simulink model "ex3"  (Simulink 6.3)
settings: Solver=VariableStepDiscrete  StartTime=0.0  StopTime=10  RelTol=1e-3
values from neighbouring files (symbols this model uses):
  SymbolRate = 50000    [ex3sim.m]
undefined symbols (not defined in the file or in its folder): gfprimfd
libraries: commdigbbndpm2 x4, dspbuff3 x3, commchan3 x2, commsink2 x2, commblkcod2 x2, dspsigops x1, commrandsrc2 x1
settings Model: LastModifiedBy=lxy  StrictBusMsg=None
settings OptimizationCC: InlineInvariantSignals=on

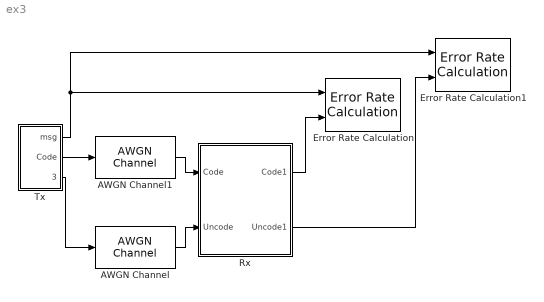
== system ex3 ==
  AWGN Channel : commchan3/AWGN Channel  seed=12345  noiseMode="Signal to noise ratio  (Eb/No)"  EbNodB=SNR  EsNodB=10  SNRdB=10  bitsPerSym=2  Ps=1  Tsym=1/SymbolRate  variance=1
  AWGN Channel1 : commchan3/AWGN Channel  seed=12345  noiseMode="Signal to noise ratio  (Eb/No)"  EbNodB=SNR  EsNodB=10  SNRdB=10  bitsPerSym=2  Ps=1  Tsym=1/SymbolRate  variance=1
  Error Rate Calculation : commsink2/Error Rate Calculation  N=8  st_delay=0  cp_mode=Entire frame  subframe=[]  PMode=Workspace  WsName=BER2  RsMode2=off  stop=off  numErr=100  maxBits=1e6
  Error Rate Calculation1 : commsink2/Error Rate Calculation  N=0  st_delay=0  cp_mode=Entire frame  subframe=[]  PMode=Workspace  WsName=BER1  RsMode2=off  stop=off  numErr=100  maxBits=1e6
  Rx : Subsystem
  Tx : Subsystem
  wires:
  Tx/2(Code) -> AWGN Channel1/1
  Tx/3(Uncode) -> AWGN Channel/1
  AWGN Channel/1 -> Rx/2(Uncode)
  AWGN Channel1/1 -> Rx/1(Code)
  Tx/1(msg) -> Error Rate Calculation/1, Error Rate Calculation1/1
  Rx/1(Code1) -> Error Rate Calculation/2
  Rx/2(Uncode1) -> Error Rate Calculation1/2

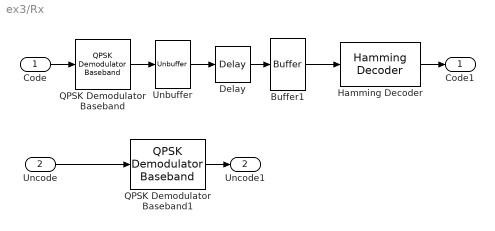
== system ex3/Rx ==
  Code : Inport
  Uncode : Inport  Port=2
  Buffer1 : dspbuff3/Buffer  N=7  V=0  ic=4
  Delay : dspsigops/Delay  dly_unit=Samples  delay=5  ic_detail=off  dif_ic_for_ch=off  dif_ic_for_dly=off  ic=0  reset_popup=None
  Hamming Decoder : commblkcod2/Hamming Decoder  n=7  k=gfprimfd(3,'min')
  QPSK Demodulator Baseband : commdigbbndpm2/QPSK Demodulator Baseband  OutType=Bit  Dec=Gray  Ph=pi/4  numSamp=1
  QPSK Demodulator Baseband1 : commdigbbndpm2/QPSK Demodulator Baseband  OutType=Bit  Dec=Gray  Ph=pi/4  numSamp=1
  Unbuffer : dspbuff3/Unbuffer  ic=0
  Code1 : Outport
  Uncode1 : Outport  Port=2
  wires:
  Hamming Decoder/1 -> Code1/1
  Code/1 -> QPSK Demodulator Baseband/1
  Uncode/1 -> QPSK Demodulator Baseband1/1
  QPSK Demodulator Baseband1/1 -> Uncode1/1
  QPSK Demodulator Baseband/1 -> Unbuffer/1
  Unbuffer/1 -> Delay/1
  Delay/1 -> Buffer1/1
  Buffer1/1 -> Hamming Decoder/1

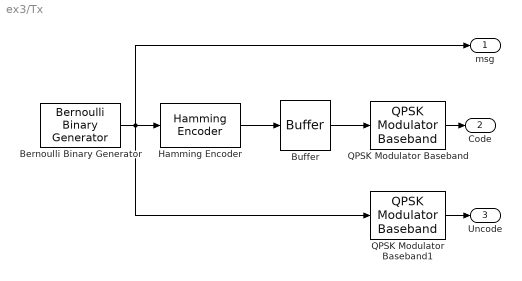
== system ex3/Tx ==
  Bernoulli Binary Generator : commrandsrc2/Bernoulli Binary Generator  P=0.5  seed=61  Ts=1/(2*SymbolRate)  frameBased=on  sampPerFrame=4  orient=off  outDataType=double
  Buffer : dspbuff3/Buffer  N=2  V=0  ic=0
  Hamming Encoder : commblkcod2/Hamming Encoder  n=7  k=gfprimfd(3,'min')
  QPSK Modulator Baseband : commdigbbndpm2/QPSK Modulator Baseband  InType=Bit  Enc=Gray  Ph=pi/4  numSamp=1
  QPSK Modulator Baseband1 : commdigbbndpm2/QPSK Modulator Baseband  InType=Bit  Enc=Gray  Ph=pi/4  numSamp=1
  msg : Outport
  Code : Outport  Port=2
  Uncode : Outport  Port=3
  wires:
  Buffer/1 -> QPSK Modulator Baseband/1
  QPSK Modulator Baseband/1 -> Code/1
  QPSK Modulator Baseband1/1 -> Uncode/1
  Bernoulli Binary Generator/1 -> Hamming Encoder/1, msg/1, QPSK Modulator Baseband1/1
  Hamming Encoder/1 -> Buffer/1
